simulink model "Tasks"  (R2024b)
settings: Solver=VariableStepAuto  StartTime=0.0  StopTime=3  RelTol=1e-3
model workspace (MATLAB code in the model file):
  | Ke = (2.53*10^(-3))*60/(2*pi); %V/(rad/s) Back EMF constant
  | Km = 24.2*10^(-3); %Nm/A    torque constant
  | L = 73*10^(-6); %H Terminal induction
  | R = 0.22; %ohm Terminal resictance
  | V = 24; %V Nominal supply voltage
  | J = 130*10^(-7);%kgm^2 %rotor inertia
  | frT = (7.72*10^(-7))*60/(2*pi); %Nm/(rad/s)  Friction torque dynamic
  | frTs=4.96e-3; %Nm Friction torque static
  | taum=4.9e-3; %Mechanical time constant
  | Mh=2635e-3; %Stall torqe Nm
  | I0=0.527; %no load current A
  | RADps_to_rpm=60/(2*pi);
  | RT=148e-3; %Rated torqe Nm
  | Rn=9650; %RPM rated speed
  | Rnnl=9700; %RPM rated speed no load
  | Mmaxout=55; %Max output torq
  | n=Mmaxout/Mh;
  | n1=n^0.5;
  | n2=n^0.5;
  | Jg1=6.5e-8;
  | Jg2=5.3e-8;
  | Jg=Jg1+(Jg2/(n1^2));
  | dj=1.5; %Nms/rad
  | 
  | dt=1.5; %Nms/rad
  | Kt=739; %Nm/rad
  | output_shaft_legth=(7.042+13.1+58)*(10^-3); %fyrkantstapp not included
  | avrage_diameter_output_shaft=(((24.5*10)+(19.6*11)+((58-19.6-24.5)*14)+(13.1*19.6)+(27.7*7.042))*(10^-6))/(output_shaft_legth); %fyrkantstapp not included.
  | input_shaft_solid_legth= (40.3-14)*10^-3;
  | avrage_diameter_input_solid_shaft= (((40.3-16.2)*5.9+(16.2-14)*11)*10^-6)/avrage_diameter_output_shaft;
  | input_shaft_hollow_legth=14e-3;
  | avrage_Odiameter_input_hollow_shaft=11e-3;
  | avrage_idiameter_input_hollow_shaft=8e-3;
  | Steel_density=7850; %kg/m^3
  | output_shaft_inertia=(Steel_density*output_shaft_legth*pi*((avrage_diameter_output_shaft/2)^4))/2;
  | input_shaft_solid_inertia=(Steel_density*input_shaft_solid_legth*pi*((avrage_diameter_input_solid_shaft/2)^4))/2;
  | input_shaft_hollow_inertia=(Steel_density*input_shaft_hollow_legth*pi*((avrage_Odiameter_input_hollow_shaft^2/4)-(avrage_idiameter_input_hollow_shaft^2/4)))*(((avrage_idiameter_input_hollow_shaft/2)^2)+((avrage_Odiameter_input_hollow_shaft/2)^2))/2;
  | input_shaft_inertia=input_shaft_hollow_inertia+input_shaft_solid_inertia;
  | Jin=input_shaft_inertia;
  | Jout=output_shaft_inertia;
  | J1=Jg+Jin+J;
  | J2=Jout;
  | A_Task6 =  [0, 0, 1, 0;
  |             0, 0, 0, 1;
  |             -Kt/(J1*n^2), Kt/(n*J1) , -(((dt/n^2)+(frT)+(Km*Ke/R))/J1),dt/(J1*n);
  |             Kt/(J2*n), -(Kt)/J2,dt/(n*J2), -(dj+dt)/J2];
  | B_Task6 = [0;
  |            0;
  |            Km/(R*J1);
  |            0];
  | C_Task6 = eye(4);
  | D_Task6 = [0;0;0;0];
  | 
  | 
  | 
  | Ks=4;%N/m
  | 
  | A_Task8 =  [0, 0, 1, 0;
  |             0, 0, 0, 1;
  |             -Kt/(J1*n^2), Kt/(n*J1) , -(((dt/n^2)+(frT)+(Km*Ke/R))/J1),dt/(J1*n);
  |             Kt/(J2*n), -(Kt+Ks)/J2,dt/(n*J2), -(dj+dt)/J2];
  | B_Task8 = [0;
  |            0;
  |            Km/(R*J1);
  |            0];
  | C_Task8 = eye(4);
  | D_Task8 = [0;0;0;0];
  | T=25;
  | Wtarget=3;
  | 
  | 
  | P=1.25e-3;%m
  | E=200e9; %Pa
  | Kj=Ks;
  | L0=100e-3; %m
  | sigmay=640e6; %Pa
  | %TargetT=(2*pi*L0*Kj*sigmay/(P*E));
  | r=4e-3; %m
  | Fy=pi*(r^2)*sigmay*10^6; %N
  | my=0.1;%-
  | Tmy=Fy*my*r; %Nm
  | thetay=(sigmay/((P/L0)*E))/(2*pi); %rad
  | Ftheta=(P/L0)*E*pi*(r^2)*2*pi*thetay*10^6; %F as a function of theta
  | Ty=Ks*thetay; %Nm
  | TargetT=Ty+Tmy; %Nm
  | 
  | 
  | Kpf=3/2.98;
undefined symbols (not defined in the file): sigbuilder_block
libraries: fl_lib x68, nesl_utility x18, slpidlib x5, sm_lib x4
(part 2 of 2)

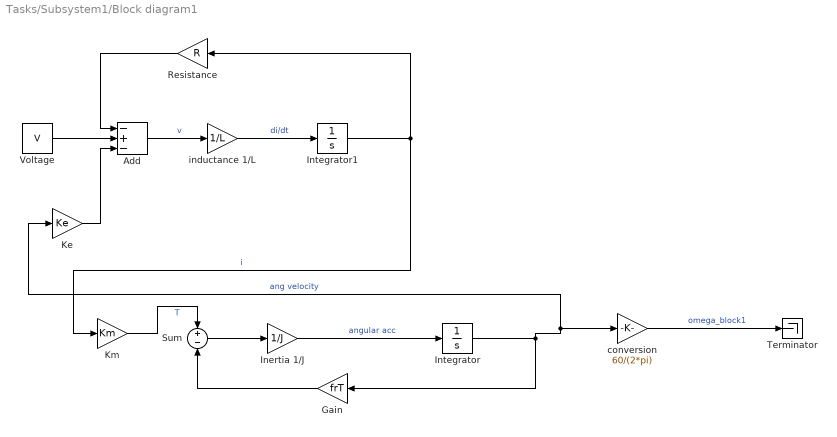
== system Tasks/Subsystem1/Block diagram1 ==
  Add : Sum  Inputs=-+-
  Gain : Gain  Gain=frT
  Inertia 1/J : Gain  Gain=1/J
  Integrator : Integrator
  Integrator1 : Integrator
  Ke : Gain  Gain=Ke
  Km : Gain  Gain=Km
  Resistance : Gain  Gain=R
  Sum : Sum  Inputs=+-
  Terminator : Terminator
  Voltage : Constant  Value=V
  conversion : Gain  Gain=60/(2*pi)
  inductance 1/L : Gain  Gain=1/L
  wires:
  Add/1 -> inductance 1/L/1  "v"
  Integrator/1 -> conversion/1, Ke/1, Gain/1  "ang velocity"
  Voltage/1 -> Add/2
  inductance 1/L/1 -> Integrator1/1  "di/dt"
  Inertia 1/J/1 -> Integrator/1  "angular acc"
  Resistance/1 -> Add/1
  Integrator1/1 -> Km/1, Resistance/1  "i"
  Sum/1 -> Inertia 1/J/1
  Gain/1 -> Sum/2
  Km/1 -> Sum/1  "T"
  Ke/1 -> Add/3
  conversion/1 -> Terminator/1  "omega_block1"

== system Tasks/Subsystem1/SD  ==
  note: Space-State Representation

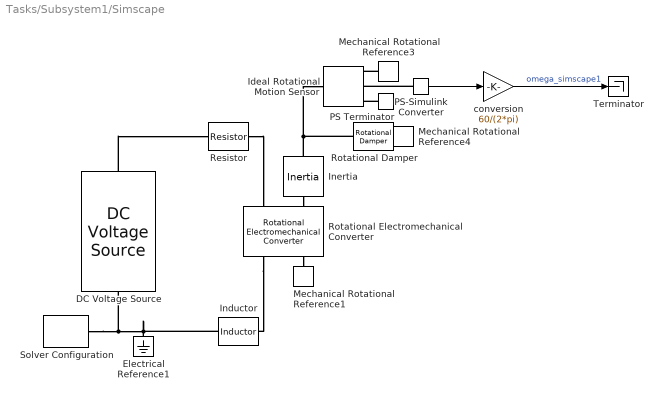
== system Tasks/Subsystem1/Simscape  ==
  DC Voltage Source : fl_lib/Electrical/Electrical Sources/DC Voltage Source  v0=V V
  Electrical Reference1 : fl_lib/Electrical/Electrical Elements/Electrical Reference
  Ideal Rotational Motion Sensor : fl_lib/Mechanical/Mechanical Sensors/Ideal Rotational Motion Sensor  reference=foundation.enum.MeasurementReference.difference  acceleration_port=false  velocity_port=true  position_port=true  wrap_angle=simscape.enum.onoff.off  offset=0 rad
  Inductor : fl_lib/Electrical/Electrical Elements/Inductor  l=L H  r=0 Ohm  g=0 1/Ohm  i_specify=off  i_priority=None  i=0 A  i_nominal_specify=off  i_nominal_value=1  i_nominal_unit=A  v_specify=off  v_priority=None  v=0 V  v_nominal_specify=off  v_nominal_value=1  v_nominal_unit=V  i_L_specify=off  i_L_priority=High  i_L=0 A  i_L_nominal_specify=off  i_L_nominal_value=1  i_L_nominal_unit=A
  Inertia : fl_lib/Mechanical/Rotational Elements/Inertia  inertia=J kg*m^2  num_ports=foundation.enum.numPorts2.two  w_specify=off  w_priority=High  w=0 rad/s  w_nominal_specify=off  w_nominal_value=1  w_nominal_unit=rad/s  t_specify=off  t_priority=None  t=0 N*m  t_nominal_specify=off  t_nominal_value=1  t_nominal_unit=N*m
      settings: InternalSimscapePortConfiguration="{\"Bottom\":[],\"Left\":[{\"id\":\"I\",\"label\":\"\",\"type\":\"foundation.mechanical.rotational.rotational\"}],\"Right\":[{\"id\":\"J\",\"label\":\"\",\"type\":\"foundation.mechanical.rotational.rotational\"}],\"Top\":[]}"
  Mechanical Rotational Reference1 : fl_lib/Mechanical/Rotational Elements/Mechanical Rotational Reference
  Mechanical Rotational Reference3 : fl_lib/Mechanical/Rotational Elements/Mechanical Rotational Reference
  Mechanical Rotational Reference4 : fl_lib/Mechanical/Rotational Elements/Mechanical Rotational Reference
  PS Terminator : fl_lib/Physical Signals/Sinks/PS Terminator
  PS-Simulink Converter : nesl_utility/PS-Simulink Converter  PhysicalDomain=network_engine_domain  SubClassName=ps_output  LeftPortType=input  RightPortType=output  PseudoPeriodic=off  Frequencies=[]  VectorFormat=inherit  Unit=inherit  AffineConversion=off
  Resistor : fl_lib/Electrical/Electrical Elements/Resistor  R=R Ohm  i_specify=off  i_priority=None  i=0 A  i_nominal_specify=off  i_nominal_value=1  i_nominal_unit=A  v_specify=off  v_priority=None  v=0 V  v_nominal_specify=off  v_nominal_value=1  v_nominal_unit=V
  Rotational Electromechanical Converter : fl_lib/Electrical/Electrical Elements/Rotational Electromechanical Converter  K=Ke V*s/rad  i_specify=off  i_priority=None  i=0 A  i_nominal_specify=off  i_nominal_value=1  i_nominal_unit=A  v_specify=off  v_priority=None  v=0 V  v_nominal_specify=off  v_nominal_value=1  v_nominal_unit=V  t_specify=off  t_priority=None  t=0 N*m  t_nominal_specify=off  t_nominal_value=1  t_nominal_unit=N*m  w_specify=on  w_priority=None  w=0 rad/s  w_nominal_specify=off  w_nominal_value=1  w_nominal_unit=rad/s
  Rotational Damper : fl_lib/Mechanical/Rotational Elements/Rotational Damper  D=frT N*m*s/rad  w_specify=off  w_priority=None  w=0 rad/s  w_nominal_specify=off  w_nominal_value=1  w_nominal_unit=rad/s  t_specify=off  t_priority=None  t=0 N*m  t_nominal_specify=off  t_nominal_value=1  t_nominal_unit=N*m
  Solver Configuration : nesl_utility/Solver Configuration  PhysicalDomain=network_engine_domain  SubClassName=solver  LeftPortType=input  RightPortType=generic  Tones=[]  Harmonics=[]  SimulateNoise=off  Profile=off  UseLocalSampling=off  EnableSwitchedLinearOptims=on  FrequencyDomain=off  UseCCode=off  RelTol=0.001  AbsTol=0.001  MinStep=1e-09  ToWorkspace=off  RevertToSquareIcSolve=off  NumHomotopyIterations=100  PhasorMode=off  PhasorModeNumHarmonics=1  ConsistencySolver=NEWTON_FTOL  IndexReductionMethod=DerivativeReplacement  DoDC=off  ResidualTolerance=1e-09  ConsistencyTolSource=GLOBAL  ConsistencyAbsTol=0.001  ConsistencyRelTol=0.001  ConsistencyTolFactor=0.001  UseLocalSolver=off  LocalSolverChoice=NE_BACKWARD_EULER_ADVANCER  ResolveIndetEquations=on  FunctionEvalNumThread=1  LocalSolverSampleTime=0.001  DoFixedCost=off  MaxNonlinIter=3  MaxModeIter=2  ComputeImpulses=off  ImpulseIterations=2  LinearAlgebra=auto  LinearAlgebraNumThread=0  EquationFormulation=NE_TIME_EF  DelaysMemoryBudget=1024  AutomaticFiltering=on  FilteringTimeConstant=0.001  PartitionStorageMethod=AS_NEEDED  PartitionMemoryBudget=1024  PartitionMethod=ROBUST  MultibodyUseLocalSolver=off  MultibodyLocalSolverChoice=ODE1  MultibodyLocalSolverSampleTime=0.001
  Terminator : Terminator
  conversion : Gain  Gain=60/(2*pi)
  wires:
  PS-Simulink Converter/1 -> conversion/1
  conversion/1 -> Terminator/1  "omega_simscape1"
  connections:
  PS Terminator/LConn1 -- Ideal Rotational Motion Sensor/RConn3
  Rotational Damper/LConn1 -- Ideal Rotational Motion Sensor/LConn1 -- Inertia/LConn1
  Solver Configuration/RConn1 -- Inductor/RConn1 -- Electrical Reference1/LConn1 -- DC Voltage Source/RConn1
  Mechanical Rotational Reference3/LConn1 -- Ideal Rotational Motion Sensor/RConn1
  Rotational Electromechanical Converter/RConn2 -- Mechanical Rotational Reference1/LConn1
  Rotational Electromechanical Converter/RConn1 -- Inductor/LConn1
  PS-Simulink Converter/LConn1 -- Ideal Rotational Motion Sensor/RConn2
  DC Voltage Source/LConn1 -- Resistor/LConn1
  Resistor/RConn1 -- Rotational Electromechanical Converter/LConn1
  Mechanical Rotational Reference4/LConn1 -- Rotational Damper/RConn1
  Inertia/RConn1 -- Rotational Electromechanical Converter/LConn2

== system Tasks/Subsystem1/Simulink Model via State-Space Representation ==
  Constant : Constant  Value=V
  State-Space : StateSpace  A=[-frT/J Km/J; -Ke/L -R/L]  B=[0; 1/L]  C=[1 0]  D=0  InitialCondition=0
  Terminator : Terminator
  conversion1 : Gain  Gain=60/(2*pi)
  wires:
  Constant/1 -> State-Space/1
  conversion1/1 -> Terminator/1  "omega_statespace1"
  State-Space/1 -> conversion1/1

== system Tasks/Subsystem1/Simulink Model via Transfer Function  ==
  Constant1 : Constant  Value=V
  Terminator1 : Terminator
  Transfer Fcn : TransferFcn  Numerator=[Km]  Denominator=[J*L (J*R+frT*L) (Km*Ke+R*frT)]
  conversion2 : Gain  Gain=60/(2*pi)
  wires:
  conversion2/1 -> Terminator1/1  "omega_transfer"
  Transfer Fcn/1 -> conversion2/1
  Constant1/1 -> Transfer Fcn/1

== system Tasks/Subsystem2/Subsystem5 ==
  Block diagram1 : Subsystem
  Constant : Constant  Value=V
  "SD " : Subsystem
  "Simscape " : Subsystem
  Simscape multibody : Subsystem
  Simulink Model via State-Space Representation : Subsystem
  "Simulink Model via Transfer Function " : Subsystem
      settings: PortSchema="{\"entries\":[{\"content\":{\"sides\":[{\"content\":{},\"type\":\"ConnectorPlacement.EquallySpacedRectSide\",\"uuid\":\"f25cfca7-2b35-4121-a35c-71a957644b44\"},{\"content\":{\"side\":\"RIGHT\"},\"type\":\"ConnectorPlacement.EquallySpacedRectSide\",\"uuid\":\"d7ca1b08-d732-40f0-a21b-b84b5cb99286\"},{\"content\":{\"connectorIds\":[\"In1\"],\"side\":\"TOP\"},\"type\":\"ConnectorPlacement.EquallySpacedRectSide\",\"uuid\":\"8734897b-0c9a-4d28-bcf3-b286a703a4f6\"}]},\"type\":\"ConnectorPlacement.EquallySpacedConnector\",\"uuid\":\"af8b9e5d-c6f5-48ad-a3a0-a633dc765a94\"}],\"packageUris\":[\"http://schema.mathworks.com/mf0/Connector/R2020b\"],\"version\":\"1.0\"}"
  Terminator{,2..6} (6 alike) : Terminator
  wires:
  Constant/1 -> Block diagram1/1(Inport), Simscape multibody/1(Inport), "Simscape "/1(Inport), "Simulink Model via Transfer Function "/1(Inport), Simulink Model via State-Space Representation/1(Inport)
  Simulink Model via State-Space Representation/1(Out1) -> Terminator/1  "2State-Space RPM"
  "Simscape "/1(Out1) -> Terminator2/1  "2Simscape RPM"
  Block diagram1/1(Out1) -> Terminator4/1  "2Block diagram RPM"
  Simscape multibody/1(Out1) -> Terminator5/1  "2Simscape multibody"
  Simulink Model via State-Space Representation/2(Out2) -> Terminator6/1  "2ang accel ss"
  "Simscape "/2(Out2) -> Terminator3/1  "2 ang accel simscape"

== system Tasks/Subsystem4/Acceleration ref. ==
  Demux : Demux  Tag=STV Demux  Outputs=2
      settings: DisplayOption=none
  FromWs : FromWorkspace  Tag=STV FromWs  VariableName=tuvar
      SigBuilderData=|
      | common.afterFinalStr = 'Extrapolate'
      | common.sampleTime = 0
      | dataSet.timeRange = [0 10]
      | dataSet.name = 'Group 1'
      | sbobj.Groups.Name = 'Group 1'
      | sbobj.Groups.Signals(1).Name = 'Signal 1'
      | sbobj.Groups.Signals(1).XData = [0 0.2 0.2 10]
      | sbobj.Groups.Signals(1).YData = [1 1 0 0]
      | sbobj.Groups.Signals(2).Name = 'Signal 2'
      | sbobj.Groups.Signals(2).XData = [0 2.8 2.8 3 3 10]
      | sbobj.Groups.Signals(2).YData = [0 0 -1 -1 0 0]
  Signal 1 : Outport  Tag=STV Outport
  Signal 2 : Outport  Tag=STV Outport  Port=2
  wires:
  Demux/1 -> Signal 1/1
  FromWs/1 -> Demux/1
  Demux/2 -> Signal 2/1

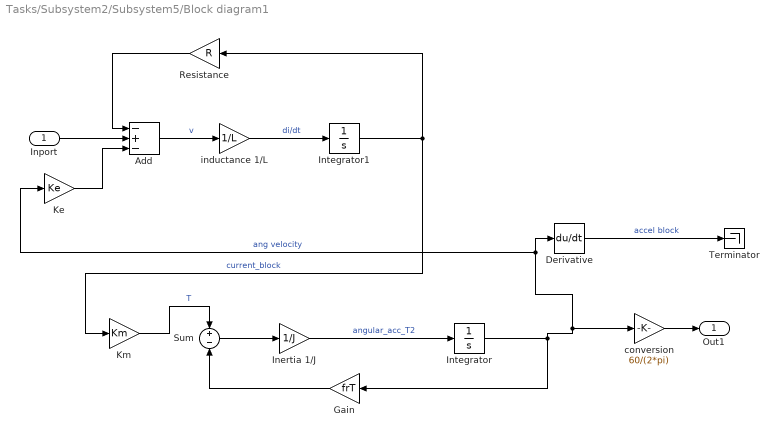
== system Tasks/Subsystem2/Subsystem5/Block diagram1 ==
  Inport : Inport
  Add : Sum  Inputs=-+-
  Derivative : Derivative
  Gain : Gain  Gain=frT
  Inertia 1/J : Gain  Gain=1/J
  Integrator : Integrator
  Integrator1 : Integrator
  Ke : Gain  Gain=Ke
  Km : Gain  Gain=Km
  Resistance : Gain  Gain=R
  Sum : Sum  Inputs=+-
  Terminator : Terminator
  conversion : Gain  Gain=60/(2*pi)
  inductance 1/L : Gain  Gain=1/L
  Out1 : Outport
  wires:
  Add/1 -> inductance 1/L/1  "v"
  Integrator/1 -> conversion/1, Derivative/1, Ke/1, Gain/1  "ang velocity"
  Inport/1 -> Add/2
  inductance 1/L/1 -> Integrator1/1  "di/dt"
  Inertia 1/J/1 -> Integrator/1  "angular_acc_T2"
  Resistance/1 -> Add/1
  Integrator1/1 -> Km/1, Resistance/1  "current_block"
  Sum/1 -> Inertia 1/J/1
  conversion/1 -> Out1/1
  Gain/1 -> Sum/2
  Km/1 -> Sum/1  "T"
  Ke/1 -> Add/3
  Derivative/1 -> Terminator/1  "accel block"

== system Tasks/Subsystem2/Subsystem5/SD  ==
  note: Space-State Representation

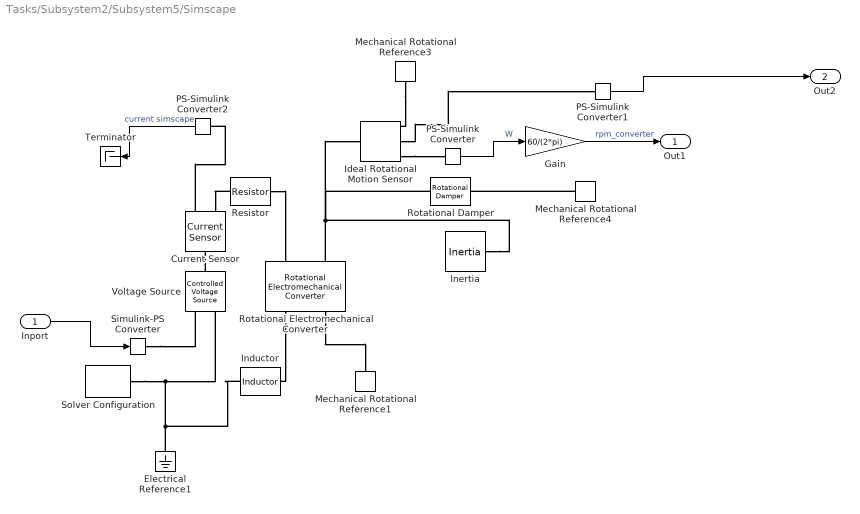
== system Tasks/Subsystem2/Subsystem5/Simscape  ==
  Inport : Inport
  Current Sensor : fl_lib/Electrical/Electrical Sensors/Current Sensor
  Electrical Reference1 : fl_lib/Electrical/Electrical Elements/Electrical Reference
  Gain : Gain  Gain=60/(2*pi)
  Ideal Rotational Motion Sensor : fl_lib/Mechanical/Mechanical Sensors/Ideal Rotational Motion Sensor  reference=foundation.enum.MeasurementReference.difference  acceleration_port=true  velocity_port=true  position_port=false  wrap_angle=simscape.enum.onoff.off  offset=0 rad
      settings: InternalSimscapePortConfiguration="{\"Bottom\":[],\"Left\":[{\"id\":\"R\",\"label\":\"R\",\"type\":\"foundation.mechanical.rotational.rotational\"}],\"Right\":[{\"id\":\"C\",\"label\":\"C\",\"type\":\"foundation.mechanical.rotational.rotational\"},{\"id\":\"alpha\",\"label\":\"α\",\"type\":\"output\"},{\"id\":\"W\",\"label\":\"W\",\"type\":\"output\"}],\"Top\":[]}"
  Inductor : fl_lib/Electrical/Electrical Elements/Inductor  l=L H  r=0 Ohm  g=0 1/Ohm  i_specify=off  i_priority=None  i=0 A  i_nominal_specify=off  i_nominal_value=1  i_nominal_unit=A  v_specify=off  v_priority=None  v=0 V  v_nominal_specify=off  v_nominal_value=1  v_nominal_unit=V  i_L_specify=off  i_L_priority=High  i_L=0 A  i_L_nominal_specify=off  i_L_nominal_value=1  i_L_nominal_unit=A
  Inertia : fl_lib/Mechanical/Rotational Elements/Inertia  inertia=J kg*m^2  num_ports=foundation.enum.numPorts2.one  w_specify=off  w_priority=High  w=0 rad/s  w_nominal_specify=off  w_nominal_value=1  w_nominal_unit=rad/s  t_specify=off  t_priority=None  t=0 N*m  t_nominal_specify=off  t_nominal_value=1  t_nominal_unit=N*m
  Mechanical Rotational Reference1 : fl_lib/Mechanical/Rotational Elements/Mechanical Rotational Reference
  Mechanical Rotational Reference3 : fl_lib/Mechanical/Rotational Elements/Mechanical Rotational Reference
  Mechanical Rotational Reference4 : fl_lib/Mechanical/Rotational Elements/Mechanical Rotational Reference
  PS-Simulink Converter : nesl_utility/PS-Simulink Converter  PhysicalDomain=network_engine_domain  SubClassName=ps_output  LeftPortType=input  RightPortType=output  PseudoPeriodic=off  Frequencies=[]  VectorFormat=inherit  Unit=inherit  AffineConversion=off
  PS-Simulink Converter1 : nesl_utility/PS-Simulink Converter  PhysicalDomain=network_engine_domain  SubClassName=ps_output  LeftPortType=input  RightPortType=output  PseudoPeriodic=off  Frequencies=[]  VectorFormat=inherit  Unit=inherit  AffineConversion=off
  PS-Simulink Converter2 : nesl_utility/PS-Simulink Converter  PhysicalDomain=network_engine_domain  SubClassName=ps_output  LeftPortType=input  RightPortType=output  PseudoPeriodic=off  Frequencies=[]  VectorFormat=inherit  Unit=inherit  AffineConversion=off
  Resistor : fl_lib/Electrical/Electrical Elements/Resistor  R=R Ohm  i_specify=off  i_priority=None  i=0 A  i_nominal_specify=off  i_nominal_value=1  i_nominal_unit=A  v_specify=off  v_priority=None  v=0 V  v_nominal_specify=off  v_nominal_value=1  v_nominal_unit=V
  Rotational Electromechanical Converter : fl_lib/Electrical/Electrical Elements/Rotational Electromechanical Converter  K=Ke V*s/rad  i_specify=off  i_priority=None  i=0 A  i_nominal_specify=off  i_nominal_value=1  i_nominal_unit=A  v_specify=off  v_priority=None  v=0 V  v_nominal_specify=off  v_nominal_value=1  v_nominal_unit=V  t_specify=off  t_priority=None  t=0 N*m  t_nominal_specify=off  t_nominal_value=1  t_nominal_unit=N*m  w_specify=on  w_priority=None  w=0 rad/s  w_nominal_specify=off  w_nominal_value=1  w_nominal_unit=rad/s
  Rotational Damper : fl_lib/Mechanical/Rotational Elements/Rotational Damper  D=frT N*m*s/rad  w_specify=off  w_priority=None  w=0 rad/s  w_nominal_specify=off  w_nominal_value=1  w_nominal_unit=rad/s  t_specify=off  t_priority=None  t=0 N*m  t_nominal_specify=off  t_nominal_value=1  t_nominal_unit=N*m
  Simulink-PS Converter : nesl_utility/Simulink-PS Converter  PhysicalDomain=network_engine_domain  SubClassName=ps_input  LeftPortType=input  RightPortType=output  PseudoPeriodic=off  Frequencies=[]  NoiseDistribution=none  NoiseParameters=[]  Unit=1  AffineConversion=off  FilteringAndDerivatives=provide  SimscapeFilterOrder=1  InputFilterTimeConstant=0.001  UdotUserProvided=0
  Solver Configuration : nesl_utility/Solver Configuration  PhysicalDomain=network_engine_domain  SubClassName=solver  LeftPortType=input  RightPortType=generic  Tones=[]  Harmonics=[]  SimulateNoise=off  Profile=off  UseLocalSampling=off  EnableSwitchedLinearOptims=on  FrequencyDomain=off  UseCCode=off  RelTol=0.001  AbsTol=0.001  MinStep=1e-09  ToWorkspace=off  RevertToSquareIcSolve=off  NumHomotopyIterations=100  PhasorMode=off  PhasorModeNumHarmonics=1  ConsistencySolver=NEWTON_FTOL  IndexReductionMethod=DerivativeReplacement  DoDC=off  ResidualTolerance=1e-09  ConsistencyTolSource=GLOBAL  ConsistencyAbsTol=0.001  ConsistencyRelTol=0.001  ConsistencyTolFactor=0.001  UseLocalSolver=off  LocalSolverChoice=NE_BACKWARD_EULER_ADVANCER  ResolveIndetEquations=on  FunctionEvalNumThread=1  LocalSolverSampleTime=0.001  DoFixedCost=off  MaxNonlinIter=3  MaxModeIter=2  ComputeImpulses=off  ImpulseIterations=2  LinearAlgebra=auto  LinearAlgebraNumThread=0  EquationFormulation=NE_TIME_EF  DelaysMemoryBudget=1024  AutomaticFiltering=on  FilteringTimeConstant=0.001  PartitionStorageMethod=AS_NEEDED  PartitionMemoryBudget=1024  PartitionMethod=ROBUST  MultibodyUseLocalSolver=off  MultibodyLocalSolverChoice=ODE1  MultibodyLocalSolverSampleTime=0.001
  Terminator : Terminator
  Voltage Source : fl_lib/Electrical/Electrical Sources/Controlled Voltage Source
  Out1 : Outport
  Out2 : Outport  Port=2
  wires:
  Gain/1 -> Out1/1  "rpm_converter"
  PS-Simulink Converter/1 -> Gain/1  "W"
  Inport/1 -> Simulink-PS Converter/1
  PS-Simulink Converter1/1 -> Out2/1
  PS-Simulink Converter2/1 -> Terminator/1  "current simscape"
  connections:
  Inertia/LConn1 -- Rotational Electromechanical Converter/LConn2 -- Rotational Damper/LConn1 -- Ideal Rotational Motion Sensor/LConn1
  Electrical Reference1/LConn1 -- Inductor/RConn1 -- Solver Configuration/RConn1 -- Voltage Source/RConn2
  Mechanical Rotational Reference3/LConn1 -- Ideal Rotational Motion Sensor/RConn1
  Rotational Electromechanical Converter/RConn2 -- Mechanical Rotational Reference1/LConn1
  Rotational Electromechanical Converter/RConn1 -- Inductor/LConn1
  Resistor/RConn1 -- Rotational Electromechanical Converter/LConn1
  Mechanical Rotational Reference4/LConn1 -- Rotational Damper/RConn1
  Simulink-PS Converter/RConn1 -- Voltage Source/RConn1
  Ideal Rotational Motion Sensor/RConn2 -- PS-Simulink Converter1/LConn1
  Ideal Rotational Motion Sensor/RConn3 -- PS-Simulink Converter/LConn1
  Resistor/LConn1 -- Current Sensor/RConn2
  Voltage Source/LConn1 -- Current Sensor/LConn1
  Current Sensor/RConn1 -- PS-Simulink Converter2/LConn1

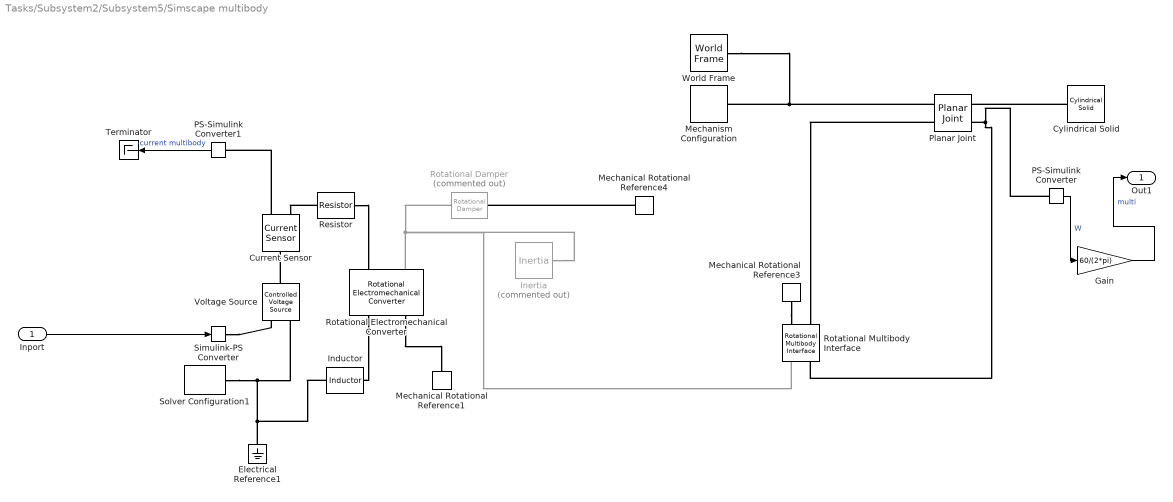
== system Tasks/Subsystem2/Subsystem5/Simscape multibody ==
  Inport : Inport
  Current Sensor : fl_lib/Electrical/Electrical Sensors/Current Sensor
  Cylindrical Solid : sm_lib/Body Elements/Cylindrical Solid  CylinderRadius=0.006  CylinderRadiusUnits=m  CylinderLength=0.02  CylinderLengthUnits=m  ExportEntireGeometry=off  InertiaType=Custom  BasedOnType=Mass  Density=1000  DensityUnits=kg/m^3  Mass=1  MassUnits=kg  CenterOfMass=[0 0 0]  CenterOfMassUnits=m  MomentsOfInertia=[0 0 J]  MomentsOfInertiaUnits=kg*m^2  ProductsOfInertia=[0 0 0]  ProductsOfInertiaUnits=kg*m^2  GraphicType=FromGeometry  MarkerShape=Sphere  MarkerSize=10  GraphicVisPropType=SimpleVisualProperties  GraphicDiffuseColor=[0.5 0.5 0.5]  GraphicOpacity=1.0  GraphicSpecularColor=[0.5 0.5 0.5 1.0]  GraphicAmbientColor=[0.15 0.15 0.15 1.0]  GraphicEmissiveColor=[0.0 0.0 0.0 1.0]  GraphicShininess=75  DoExposeReferenceFrame=on  SerializedFrames=<Frames><Frame><Id>Frame1</Id><Value><Name>F1</Name><Origin><Source>ReferenceFrame</Source><FeatureName></FeatureName></Origin><PrimaryAxis><DefinedDirection>+Z</DefinedDirection><Source>ReferenceFrame</Source><SourceDirection>+Z</SourceDirection><FeatureName></FeatureName></PrimaryAxis><SecondaryAxis><DefinedDirection>+X</DefinedDirection><Source>ReferenceFrame</Source><SourceDirection>+X</SourceDirection><FeatureName></FeatureName></SecondaryAxis></Value></Frame></Frames>
  Electrical Reference1 : fl_lib/Electrical/Electrical Elements/Electrical Reference
  Gain : Gain  Gain=60/(2*pi)
  Inductor : fl_lib/Electrical/Electrical Elements/Inductor  l=L H  r=0 Ohm  g=0 1/Ohm  i_specify=off  i_priority=None  i=0 A  i_nominal_specify=off  i_nominal_value=1  i_nominal_unit=A  v_specify=off  v_priority=None  v=0 V  v_nominal_specify=off  v_nominal_value=1  v_nominal_unit=V  i_L_specify=off  i_L_priority=High  i_L=0 A  i_L_nominal_specify=off  i_L_nominal_value=1  i_L_nominal_unit=A
  Inertia : fl_lib/Mechanical/Rotational Elements/Inertia  Commented=on  inertia=J kg*m^2  num_ports=foundation.enum.numPorts2.one  w_specify=off  w_priority=High  w=0 rad/s  w_nominal_specify=off  w_nominal_value=1  w_nominal_unit=rad/s  t_specify=off  t_priority=None  t=0 N*m  t_nominal_specify=off  t_nominal_value=1  t_nominal_unit=N*m
  Mechanical Rotational Reference1 : fl_lib/Mechanical/Rotational Elements/Mechanical Rotational Reference
  Mechanical Rotational Reference3 : fl_lib/Mechanical/Rotational Elements/Mechanical Rotational Reference
  Mechanical Rotational Reference4 : fl_lib/Mechanical/Rotational Elements/Mechanical Rotational Reference
  Mechanism Configuration : sm_lib/Utilities/Mechanism Configuration  UniformGravity=Constant  GravityVector=[0 0 -9.80665]  GravityVectorUnits=m/s^2  LinearizationDelta=0.001  JointModeTransitionNonlinearIterations=2
  PS-Simulink Converter : nesl_utility/PS-Simulink Converter  PhysicalDomain=network_engine_domain  SubClassName=ps_output  LeftPortType=input  RightPortType=output  PseudoPeriodic=off  Frequencies=[]  VectorFormat=inherit  Unit=inherit  AffineConversion=off
  PS-Simulink Converter1 : nesl_utility/PS-Simulink Converter  PhysicalDomain=network_engine_domain  SubClassName=ps_output  LeftPortType=input  RightPortType=output  PseudoPeriodic=off  Frequencies=[]  VectorFormat=inherit  Unit=inherit  AffineConversion=off
  Planar Joint : sm_lib/Joints/Planar Joint  JointMode=Normal  CompositeWrenchDir=FollowerOnBase  CompositeWrenchFrame=BaseFrame  SenseConstraintForce=off  SenseConstraintTorque=off  SenseTotalForce=off  SenseTotalTorque=off  PxPositionTargetSpecify=on  PxPositionTargetPriority=High  PxPositionTargetValue=0  PxPositionTargetValueUnits=m  PxVelocityTargetSpecify=on  PxVelocityTargetPriority=High  PxVelocityTargetValue=0  PxVelocityTargetValueUnits=m/s  PxEquilibriumPosition=0  PxEquilibriumPositionUnits=m  PxSpringStiffness=0  PxSpringStiffnessUnits=N/m  PxDampingCoefficient=0  PxDampingCoefficientUnits=N/(m/s)  PxLowerLimitSpecify=off  PxLowerLimitBound=-1  PxLowerLimitBoundUnits=m  PxLowerLimitStiffness=1e6  PxLowerLimitStiffnessUnits=N/m  PxLowerLimitDamping=1e3  PxLowerLimitDampingUnits=N/(m/s)  PxLowerLimitTransitionRegionWidth=1e-4  PxLowerLimitTransitionRegionWidthUnits=m  PxUpperLimitSpecify=off  PxUpperLimitBound=1  PxUpperLimitBoundUnits=m  PxUpperLimitStiffness=1e6  PxUpperLimitStiffnessUnits=N/m  PxUpperLimitDamping=1e3  PxUpperLimitDampingUnits=N/(m/s)  PxUpperLimitTransitionRegionWidth=1e-4  PxUpperLimitTransitionRegionWidthUnits=m  PxTorqueActuationMode=NoTorque  PxMotionActuationMode=ComputedMotion  PxSensePosition=off  PxSenseVelocity=off  PxSenseAcceleration=off  PxSenseTorqueForce=off  PxSenseLowerLimitTorqueForce=off  PxSenseUpperLimitTorqueForce=off  PyPositionTargetSpecify=off  PyPositionTargetPriority=High  PyPositionTargetValue=0  PyPositionTargetValueUnits=m  PyVelocityTargetSpecify=off  PyVelocityTargetPriority=High  PyVelocityTargetValue=0  PyVelocityTargetValueUnits=m/s  PyEquilibriumPosition=0  PyEquilibriumPositionUnits=m  PySpringStiffness=0  PySpringStiffnessUnits=N/m  PyDampingCoefficient=0  PyDampingCoefficientUnits=N/(m/s)  PyLowerLimitSpecify=off  PyLowerLimitBound=-1  PyLowerLimitBoundUnits=m  PyLowerLimitStiffness=1e6  PyLowerLimitStiffnessUnits=N/m  PyLowerLimitDamping=1e3  PyLowerLimitDampingUnits=N/(m/s)  PyLowerLimitTransitionRegionWidth=1e-4  PyLowerLimitTransitionRegionWidthUnits=m  PyUpperLimitSpecify=off  PyUpperLimitBound=1  PyUpperLimitBoundUnits=m  PyUpperLimitStiffness=1e6  PyUpperLimitStiffnessUnits=N/m  PyUpperLimitDamping=1e3  PyUpperLimitDampingUnits=N/(m/s)  PyUpperLimitTransitionRegionWidth=1e-4  PyUpperLimitTransitionRegionWidthUnits=m  PyTorqueActuationMode=NoTorque  PyMotionActuationMode=ComputedMotion  PySensePosition=off  PySenseVelocity=off  PySenseAcceleration=off  PySenseTorqueForce=off  PySenseLowerLimitTorqueForce=off  PySenseUpperLimitTorqueForce=off  RzPositionTargetSpecify=off  RzPositionTargetPriority=High  RzPositionTargetValue=0  RzPositionTargetValueUnits=deg  RzVelocityTargetSpecify=off  RzVelocityTargetPriority=High  RzVelocityTargetValue=0  RzVelocityTargetValueUnits=deg/s  RzEquilibriumPosition=0  RzEquilibriumPositionUnits=deg  RzSpringStiffness=0  RzSpringStiffnessUnits=N*m/deg  RzDampingCoefficient=frT  RzDampingCoefficientUnits=N*m/(rad/s)  RzLowerLimitSpecify=off  RzLowerLimitBound=-90  RzLowerLimitBoundUnits=deg  RzLowerLimitStiffness=1e4  RzLowerLimitStiffnessUnits=N*m/deg  RzLowerLimitDamping=10  RzLowerLimitDampingUnits=N*m/(deg/s)  RzLowerLimitTransitionRegionWidth=0.1  RzLowerLimitTransitionRegionWidthUnits=deg  RzUpperLimitSpecify=off  RzUpperLimitBound=90  RzUpperLimitBoundUnits=deg  RzUpperLimitStiffness=1e4  RzUpperLimitStiffnessUnits=N*m/deg  RzUpperLimitDamping=10  RzUpperLimitDampingUnits=N*m/(deg/s)  RzUpperLimitTransitionRegionWidth=0.1  RzUpperLimitTransitionRegionWidthUnits=deg  RzTorqueActuationMode=InputTorque  RzMotionActuationMode=ComputedMotion  RzSensePosition=off  RzSenseVelocity=on  RzSenseAcceleration=off  RzSenseTorqueForce=off  RzSenseLowerLimitTorqueForce=off  RzSenseUpperLimitTorqueForce=off
  Resistor : fl_lib/Electrical/Electrical Elements/Resistor  R=R Ohm  i_specify=off  i_priority=None  i=0 A  i_nominal_specify=off  i_nominal_value=1  i_nominal_unit=A  v_specify=off  v_priority=None  v=0 V  v_nominal_specify=off  v_nominal_value=1  v_nominal_unit=V
  Rotational Electromechanical Converter : fl_lib/Electrical/Electrical Elements/Rotational Electromechanical Converter  K=Ke V*s/rad  i_specify=off  i_priority=None  i=0 A  i_nominal_specify=off  i_nominal_value=1  i_nominal_unit=A  v_specify=off  v_priority=None  v=0 V  v_nominal_specify=off  v_nominal_value=1  v_nominal_unit=V  t_specify=off  t_priority=None  t=0 N*m  t_nominal_specify=off  t_nominal_value=1  t_nominal_unit=N*m  w_specify=on  w_priority=None  w=0 rad/s  w_nominal_specify=off  w_nominal_value=1  w_nominal_unit=rad/s
  Rotational Damper : fl_lib/Mechanical/Rotational Elements/Rotational Damper  Commented=on  D=frT N*m*s/rad  w_specify=off  w_priority=None  w=0 rad/s  w_nominal_specify=off  w_nominal_value=1  w_nominal_unit=rad/s  t_specify=off  t_priority=None  t=0 N*m  t_nominal_specify=off  t_nominal_value=1  t_nominal_unit=N*m
  Rotational Multibody Interface : fl_lib/Mechanical/Multibody Interfaces/Rotational Multibody Interface
  Simulink-PS Converter : nesl_utility/Simulink-PS Converter  PhysicalDomain=network_engine_domain  SubClassName=ps_input  LeftPortType=input  RightPortType=output  PseudoPeriodic=off  Frequencies=[]  NoiseDistribution=none  NoiseParameters=[]  Unit=1  AffineConversion=off  FilteringAndDerivatives=provide  SimscapeFilterOrder=1  InputFilterTimeConstant=0.001  UdotUserProvided=0
  Solver Configuration1 : nesl_utility/Solver Configuration  PhysicalDomain=network_engine_domain  SubClassName=solver  LeftPortType=input  RightPortType=generic  Tones=[]  Harmonics=[]  SimulateNoise=off  Profile=off  UseLocalSampling=off  EnableSwitchedLinearOptims=on  FrequencyDomain=off  UseCCode=off  RelTol=0.001  AbsTol=0.001  MinStep=1e-09  ToWorkspace=off  RevertToSquareIcSolve=off  NumHomotopyIterations=100  PhasorMode=off  PhasorModeNumHarmonics=1  ConsistencySolver=NEWTON_FTOL  IndexReductionMethod=DerivativeReplacement  DoDC=off  ResidualTolerance=1e-09  ConsistencyTolSource=GLOBAL  ConsistencyAbsTol=0.001  ConsistencyRelTol=0.001  ConsistencyTolFactor=0.001  UseLocalSolver=off  LocalSolverChoice=NE_BACKWARD_EULER_ADVANCER  ResolveIndetEquations=on  FunctionEvalNumThread=1  LocalSolverSampleTime=0.001  DoFixedCost=off  MaxNonlinIter=3  MaxModeIter=2  ComputeImpulses=off  ImpulseIterations=2  LinearAlgebra=auto  LinearAlgebraNumThread=0  EquationFormulation=NE_TIME_EF  DelaysMemoryBudget=1024  AutomaticFiltering=on  FilteringTimeConstant=0.001  PartitionStorageMethod=AS_NEEDED  PartitionMemoryBudget=1024  PartitionMethod=ROBUST  MultibodyUseLocalSolver=off  MultibodyLocalSolverChoice=ODE1  MultibodyLocalSolverSampleTime=0.001
  Terminator : Terminator
  Voltage Source : fl_lib/Electrical/Electrical Sources/Controlled Voltage Source
  World Frame : sm_lib/Frames and Transforms/World Frame
  Out1 : Outport
  wires:
  Gain/1 -> Out1/1  "multi"
  PS-Simulink Converter/1 -> Gain/1  "W"
  Inport/1 -> Simulink-PS Converter/1
  PS-Simulink Converter1/1 -> Terminator/1  "current multibody"
  connections:
  Rotational Damper/LConn1 -- Rotational Electromechanical Converter/LConn2 -- Rotational Multibody Interface/RConn2 -- Inertia/LConn1
  PS-Simulink Converter/LConn1 -- Rotational Multibody Interface/RConn1 -- Planar Joint/RConn2
  Cylindrical Solid/LConn1 -- Planar Joint/RConn1
  Mechanical Rotational Reference3/LConn1 -- Rotational Multibody Interface/LConn2
  World Frame/RConn1 -- Planar Joint/LConn1 -- Mechanism Configuration/RConn1
  Electrical Reference1/LConn1 -- Inductor/RConn1 -- Solver Configuration1/RConn1 -- Voltage Source/RConn2
  Planar Joint/LConn2 -- Rotational Multibody Interface/LConn1
  Resistor/RConn1 -- Rotational Electromechanical Converter/LConn1
  Mechanical Rotational Reference4/LConn1 -- Rotational Damper/RConn1
  Rotational Electromechanical Converter/RConn1 -- Inductor/LConn1
  Rotational Electromechanical Converter/RConn2 -- Mechanical Rotational Reference1/LConn1
  Simulink-PS Converter/RConn1 -- Voltage Source/RConn1
  Voltage Source/LConn1 -- Current Sensor/LConn1
  Resistor/LConn1 -- Current Sensor/RConn2
  Current Sensor/RConn1 -- PS-Simulink Converter1/LConn1

== system Tasks/Subsystem2/Subsystem5/Simulink Model via State-Space Representation ==
  Inport : Inport
  Derivative : Derivative
  State-Space : StateSpace  A=[-frT/J Km/J; -Ke/L -R/L]  B=[0; 1/L]  C=[1 0]  D=0  InitialCondition=0
  conversion1 : Gain  Gain=RADps_to_rpm
  Out1 : Outport
  Out2 : Outport  Port=2
  wires:
  Inport/1 -> State-Space/1
  conversion1/1 -> Out1/1
  State-Space/1 -> Derivative/1, conversion1/1
  Derivative/1 -> Out2/1

== system Tasks/Subsystem2/Subsystem5/Simulink Model via Transfer Function  ==
  Inport : Inport
  Derivative : Derivative
  Gain : Gain  Gain=Ke/L
  Integrator : Integrator
  Terminator : Terminator
  Terminator1 : Terminator
  Transfer Fcn : TransferFcn  Numerator=[Km]  Denominator=[J*L (J*R+frT*L) (Km*Ke+R*frT)]
  wires:
  Transfer Fcn/1 -> Gain/1, Derivative/1  "trasnfer rad/s"
  Inport/1 -> Transfer Fcn/1
  Derivative/1 -> Terminator1/1  "accell transfer"
  Gain/1 -> Integrator/1
  Integrator/1 -> Terminator/1  "current transfer"
